simulink model "WaterTankSysControlPID2018"  (R2015b)
settings: Solver=FixedStepAuto  StartTime=0.0  StopTime=5*140*0.75  FixedStep=0.75  RelTol=1e-3
values from neighbouring files (symbols this model uses):
  u_offset = u_act(1)    [lab5.m]    (also in matlab.mat = 2.05)
  y_offset = mean(y_act(1:count))    [lab5.m]    (also in matlab.mat = 2.34175388168)
undefined symbols (not defined in the file or in its folder): MIO, National_Instruments, PCI
libraries: sldrtlib x4, simulink x2
settings Model: SimulationMode=external  ExtModeTrigDuration=7200  ExtModeArchiveMode=auto  ExtModeArchiveFileName=SFControlData  ExtModeArchiveDirName=C:\Users\My Project\Documents\MATLAB  ExtModeAutoIncOneShot=on  ExtModeWriteAllDataToWs=on  Creator=My Project  LastModifiedBy=My Project
settings HardwareCC: ProdBitPerLong=64  ProdLargestAtomicFloat=None  ProdHWDeviceType=Intel->x86-64  TargetBitPerLong=64  TargetBitPerPointer=64  TargetIntDivRoundTo=Zero  TargetEndianess=LittleEndian  TargetWordSize=64  TargetHWDeviceType=Intel->x86-64
settings RTWCC: SystemTargetFile=sldrt.tlc  TemplateMakefile=sldrt.tmf  Description=Simulink Desktop Real-Time  RTWCompilerOptimization=on
settings CodeAppCC: MaxIdLength=95
settings SimulinkDesktopRealTimeCC: TargetPreCompLibLocation=C:\Program Files\MATLAB\R2015b\toolbox\sldrt\lib\win64  TargetLangStandard=C89/C90 (ANSI)  SupportVariableSizeSignals=off

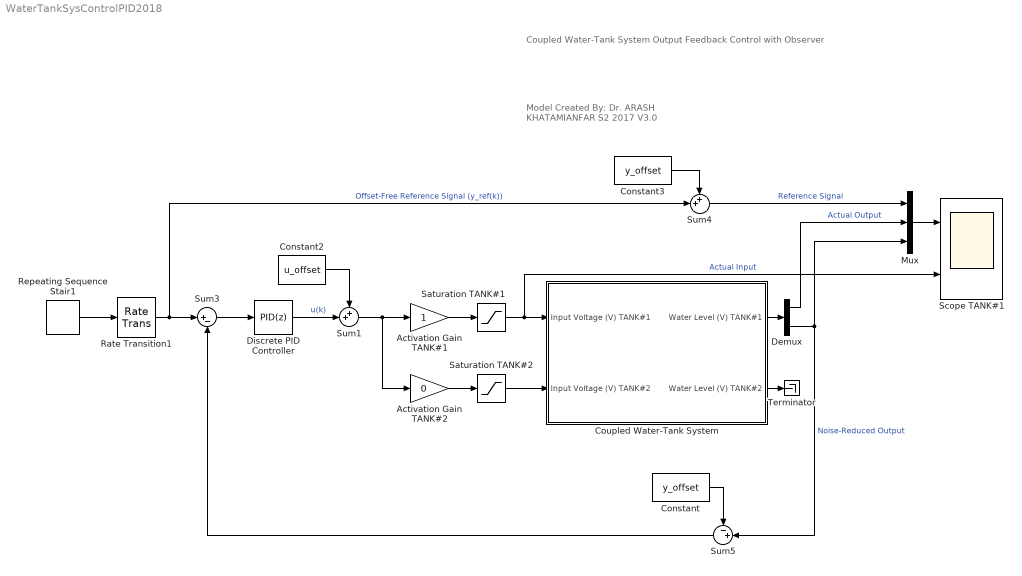
== system WaterTankSysControlPID2018 ==
  note: Model Created By:
      | Dr. ARASH KHATAMIANFAR
      | S2 2017 V3.0
  note: Coupled Water-Tank System
      | Output Feedback Control with Observer
  Activation Gain TANK#1 : Gain
  Activation Gain TANK#2 : Gain  Gain=0
  Constant : Constant  Value=y_offset
  Constant2 : Constant  Value=u_offset  SampleTime=0.75
  Constant3 : Constant  Value=y_offset  SampleTime=0.75
  Coupled Water-Tank System : Subsystem
  Demux : Demux  Outputs=2
  Discrete PID Controller : simulink/Continuous/PID Controller  Controller=PID  TimeDomain=Discrete-time  SampleTime=0.75  IntegratorMethod=Forward Euler  FilterMethod=Forward Euler  Form=Parallel  UseFilter=on  ControllerParametersSource=internal  P=0.5  I=0.02  D=0  N=100  InitialConditionSource=internal  InitialConditionForIntegrator=0  InitialConditionForFilter=0  ExternalReset=none  LimitOutput=off  UpperSaturationLimit=inf  LowerSaturationLimit=-inf  LinearizeAsGain=off  AntiWindupMode=none  Kb=1  TrackingMode=off  Kt=1  PParamMin=[]  PParamMax=[]  IParamMin=[]  IParamMax=[]  DParamMin=[]  DParamMax=[]  NParamMin=[]  NParamMax=[]  KbParamMin=[]  KbParamMax=[]  KtParamMin=[]  KtParamMax=[]  POutMin=[]  POutMax=[]  IOutMin=[]  IOutMax=[]  DOutMin=[]  DOutMax=[]  NOutMin=[]  NOutMax=[]  KbOutMin=[]  KbOutMax=[]  KtOutMin=[]  KtOutMax=[]  IntegratorOutMin=[]  IntegratorOutMax=[]  FilterOutMin=[]  FilterOutMax=[]  SumOutMin=[]  SumOutMax=[]  SumI1OutMin=[]  SumI1OutMax=[]  SumI2OutMin=[]  SumI2OutMax=[]  SumI3OutMin=[]  SumI3OutMax=[]  SumDOutMin=[]  SumDOutMax=[]  SaturationOutMin=[]  SaturationOutMax=[]  IntegratorContinuousStateAttributes=''  IntegratorStateMustResolveToSignalObject=off  IntegratorRTWStateStorageClass=Auto  FilterContinuousStateAttributes=''  FilterStateMustResolveToSignalObject=off  FilterRTWStateStorageClass=Auto  DifferentiatorICPrevScaledInput=0  DifferentiatorOutMin=[]  DifferentiatorOutMax=[]
  Mux : Mux  Inputs=3
  Rate Transition1 : RateTransition  OutPortSampleTime=0.75
  Repeating Sequence Stair1 : simulink/Sources/Repeating Sequence Stair  OutValues=[0.7 0.2 -0.5 0].'  tsamp=140*0.75  OutMin=[]  OutMax=[]  OutDataTypeStr=double  OutputDataTypeScalingMode=double  OutDataType=fixdt(0,8)  ConRadixGroup=Best Precision: Vector-wise  OutScaling=2^-12
  Saturation TANK#1 : Saturate  UpperLimit=2.5  LowerLimit=1.5
  Saturation TANK#2 : Saturate  UpperLimit=5  LowerLimit=0
  Scope TANK#1 : Scope  NumInputPorts=2
  Sum1 : Sum  Inputs=++|
  Sum3 : Sum  Inputs=|+-
  Sum4 : Sum  Inputs=++|
  Sum5 : Sum  Inputs=-+|
  Terminator : Terminator
  wires:
  Activation Gain TANK#1/1 -> Saturation TANK#1/1
  Activation Gain TANK#2/1 -> Saturation TANK#2/1
  Saturation TANK#2/1 -> Coupled Water-Tank System/2(Input Voltage (V) TANK#2)
  Sum1/1 -> Activation Gain TANK#2/1, Activation Gain TANK#1/1
  Coupled Water-Tank System/2(Water Level (V) TANK#2) -> Terminator/1
  Constant2/1 -> Sum1/1
  Sum3/1 -> Discrete PID Controller/1
  Sum5/1 -> Sum3/2
  Constant/1 -> Sum5/1
  Rate Transition1/1 -> Sum3/1, Sum4/2  "Offset-Free Reference Signal (y_ref(k))"
  Repeating Sequence Stair1/1 -> Rate Transition1/1
  Constant3/1 -> Sum4/1
  Sum4/1 -> Mux/1  "Reference Signal"
  Mux/1 -> Scope TANK#1/1
  Saturation TANK#1/1 -> Coupled Water-Tank System/1(Input Voltage (V) TANK#1), Scope TANK#1/2  "Actual Input"
  Coupled Water-Tank System/1(Water Level (V) TANK#1) -> Demux/1
  Demux/1 -> Mux/2  "Actual Output"
  Demux/2 -> Sum5/2, Mux/3  "Noise-Reduced Output"
  Discrete PID Controller/1 -> Sum1/2  "u(k)"

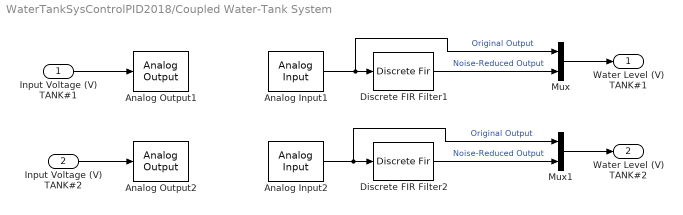
== system WaterTankSysControlPID2018/Coupled Water-Tank System ==
  Input Voltage (V) TANK#1 : Inport
  Input Voltage (V) TANK#2 : Inport  Port=2
  Analog Input1 : sldrtlib/Analog Input  SampleTime=0.75  MaxMissedTicks=10  ShowMissedTicks=off  YieldWhenWaiting=off  DrvName=National_Instruments/PCI-MIO-16E-4  DrvAddress=4294967295  DrvOptions=[0 0 0 0 0 0]  Channels=1  RangeMode=1  VoltRange=1  DataType=1
      settings: AttributesFormatString=National Instruments\nPCI-MIO-16E-4 [auto]
  Analog Input2 : sldrtlib/Analog Input  SampleTime=0.75  MaxMissedTicks=10  ShowMissedTicks=off  YieldWhenWaiting=off  DrvName=National_Instruments/PCI-MIO-16E-4  DrvAddress=4294967295  DrvOptions=[0 0 0 0 0 0]  Channels=2  RangeMode=1  VoltRange=1  DataType=1
      settings: AttributesFormatString=National Instruments\nPCI-MIO-16E-4 [auto]
  Analog Output1 : sldrtlib/Analog Output  SampleTime=0.75  MaxMissedTicks=10  ShowMissedTicks=off  YieldWhenWaiting=off  DrvName=National_Instruments/PCI-MIO-16E-4  DrvAddress=4294967295  DrvOptions=[0 0 0 0 0 0]  Channels=1  RangeMode=1  VoltRange=1  InitialValue=0  FinalValue=0
      settings: AttributesFormatString=National Instruments\nPCI-MIO-16E-4 [auto]
  Analog Output2 : sldrtlib/Analog Output  SampleTime=0.75  MaxMissedTicks=10  ShowMissedTicks=off  YieldWhenWaiting=off  DrvName=National_Instruments/PCI-MIO-16E-4  DrvAddress=4294967295  DrvOptions=[0 0 0 0 0 0]  Channels=2  RangeMode=1  VoltRange=1  InitialValue=0  FinalValue=0
      settings: AttributesFormatString=National Instruments\nPCI-MIO-16E-4 [auto]
  Discrete FIR Filter1 : DiscreteFir  Coefficients=[0.2 0.2 0.2 0.2 0.2]  SampleTime=0.75
  Discrete FIR Filter2 : DiscreteFir  Coefficients=[0.2 0.2 0.2 0.2 0.2]  SampleTime=0.75
  Mux : Mux  Inputs=2
  Mux1 : Mux  Inputs=2
  Water Level (V) TANK#1 : Outport
  Water Level (V) TANK#2 : Outport  Port=2
  wires:
  Analog Input1/1 -> Mux/1, Discrete FIR Filter1/1  "Original Output"
  Input Voltage (V) TANK#1/1 -> Analog Output1/1
  Discrete FIR Filter1/1 -> Mux/2  "Noise-Reduced Output"
  Mux/1 -> Water Level (V) TANK#1/1
  Analog Input2/1 -> Mux1/1, Discrete FIR Filter2/1  "Original Output"
  Input Voltage (V) TANK#2/1 -> Analog Output2/1
  Discrete FIR Filter2/1 -> Mux1/2  "Noise-Reduced Output"
  Mux1/1 -> Water Level (V) TANK#2/1
